simulink model "project2_sim"  (R2021b)
settings: Solver=VariableStepAuto  StartTime=0.0  StopTime=1370
values from neighbouring files (symbols this model uses):
  c0 = 0.1    [project2.m]
  c1 = 0.02    [project2.m]
  cd = 0.3    [project2.m]
  eff = 0.93    [project2.m]
  fuelmap = importdata("FuelMapLookup.csv")    [project2.m]
  G_fd = 3.36    [project2.m]
  Gear_ratio_1 = 4.58    [project2.m]
  Gear_ratio_2 = 2.96    [project2.m]
  Gear_ratio_3 = 1.91    [project2.m]
  Gear_ratio_4 = 1.45    [project2.m]
  Gear_ratio_5 = 1.00    (= 1)    [project2.m]
  Gear_ratio_6 = 0.75    [project2.m]
  input_speed = fuelmapinputs(:,2)    [project2.m]
  input_torques = fuelmapinputs(:,1)    [project2.m]
  Je = 0.1301    [project2.m]
  kd = 0.0    (= 0)    [project2.m]
  kfactor = importdata("k_factor.csv")    [project2.m]
  ki = 0.1    [project2.m]
  kp = 2.86    [project2.m]
  lower_rpm = lower_curve(:,2)    [project2.m]
  lower_torque = lower_curve(:,1)    [project2.m]
  m = (3900*.45359237)    (= 1769.010243)    [project2.m]
  max_break_torque = 375*12*2*3.36    (= 30240)    [project2.m]
  mT = 375    [project2.m]
  r = (0.339)    (= 0.339)    [project2.m]
  rho = 1.225    [project2.m]
  S = 2.3    [project2.m]
  sr = importdata("speed_ratio.csv")    [project2.m]
  time = highway(:,1)    [project2.m]
  tr = importdata("torque_ratio.csv")    [project2.m]
  upper_rpm = upper_curve(:,2)    [project2.m]
  upper_torque = upper_curve(:,1)    [project2.m]
  vel = highway(:,2)    [project2.m]
  w_idle = 720    [project2.m]
  w_max = 6400    [project2.m]
libraries: simulink x2, slpidlib x1
settings Model: Creator=franc  LastModifiedBy=franc

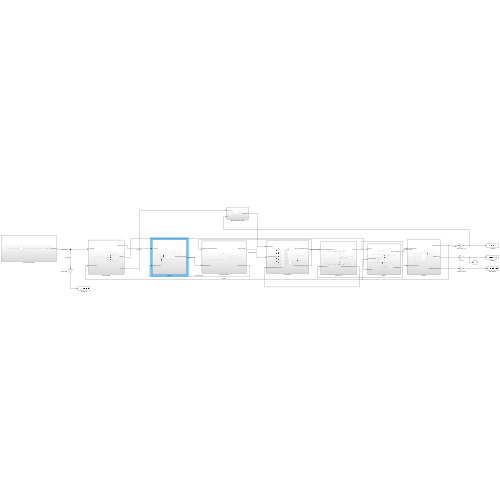
[thumbnail: Simulink's stored preview of the top-level diagram]
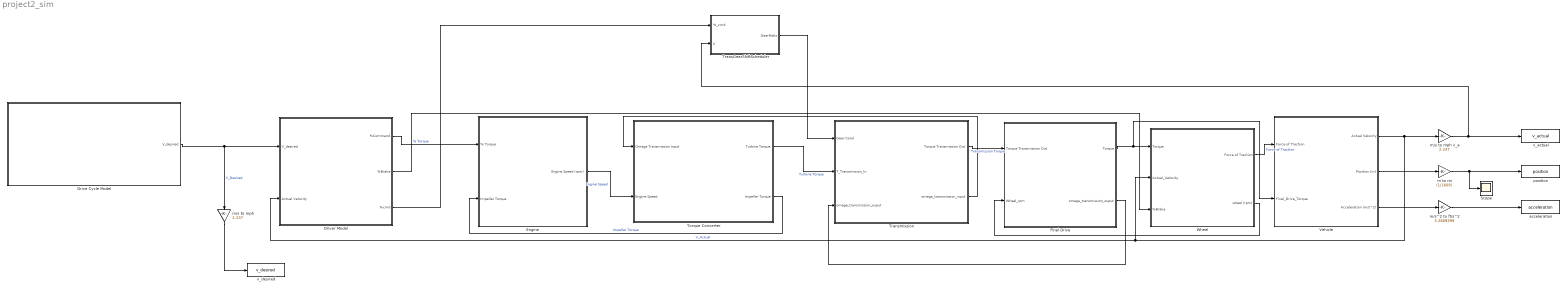
== system project2_sim ==
  " Engine" : Subsystem
  Drive Cycle Model : Subsystem
  Driver Model : Subsystem
  FInal Drive : Subsystem
  Scope : Scope
  Torque Converter : Subsystem
  TransGearShiftScheduler : Subsystem
  Transmission : Subsystem
  Vehicle : Subsystem
  Wheel : Subsystem
  acceleration : ToWorkspace  VariableName=acceleration  SaveFormat=Timeseries  SampleTime=-1
  m to mi : Gain  Gain=(1/1609)
  m/s to mph : Gain  Gain=2.237
  m/s to mph v_a : Gain  Gain=2.237
  m/s^2 to ft/s^2 : Gain  Gain=3.2808399
  position : ToWorkspace  VariableName=position  SaveFormat=Timeseries  SampleTime=-1
  v_actual : ToWorkspace  VariableName=v_actual  SaveFormat=Timeseries  SampleTime=-1
  v_desired : ToWorkspace  VariableName=v_desired  SaveFormat=Timeseries  SampleTime=-1
  wires:
  m/s to mph/1 -> v_desired/1
  m/s^2 to ft/s^2/1 -> acceleration/1
  Vehicle/1(Actual Velocity) -> Driver Model/2(Actual Velocity), Wheel/2(Actual_Velocity), m/s to mph v_a/1  "V_Actual"
  Drive Cycle Model/1(V_desired) -> m/s to mph/1, Driver Model/1(V_desired)  "V_Desired"
  Wheel/1(Force of Traction) -> Vehicle/1(Force of Traction)  "Force of Traction"
  Vehicle/2(Position (m)) -> m to mi/1
  Vehicle/3(Acceleration (m/s^2)) -> m/s^2 to ft/s^2/1
  m to mi/1 -> Scope/1, position/1
  Driver Model/1(%Command) -> " Engine"/1(% Torque)  "% Torque"
  Torque Converter/1(Turbine Torque) -> Transmission/2(T_Transmission_In)  "Turbine Torque"
  Transmission/2(omega_transmission_input) -> Torque Converter/1(Omega Transmission Input)
  Torque Converter/2(Impeller Torque) -> " Engine"/2(Impeller Torque)  "Impeller Torque"
  " Engine"/1(Engine Speed (rpm)) -> Torque Converter/2(Engine Speed)  "Engine Speed"
  m/s to mph v_a/1 -> TransGearShiftScheduler/2(V), v_actual/1
  TransGearShiftScheduler/1(GearRatio) -> Transmission/1(Gear Cond)
  Driver Model/2(%Brake) -> Wheel/3(%Brake)
  Driver Model/3(%cmd) -> TransGearShiftScheduler/1("%_cmd ")
  Transmission/1(Torque Transmission Out) -> FInal Drive/1(Torque Transmission Out)  "Transmission Torque"
  Wheel/2(wheel (rpm)) -> FInal Drive/2(Wheel_rpm)
  FInal Drive/2(omega_transmission_ouput) -> Transmission/3(omega_transmission_ouput)
  FInal Drive/1(Torque) -> Wheel/1(Torque), Vehicle/2(Final_Drive_Torque)

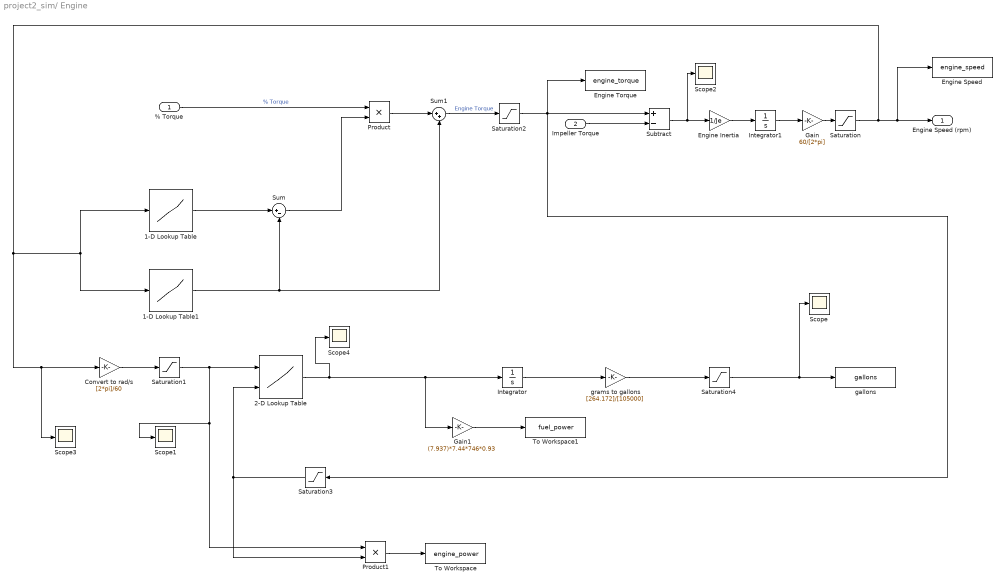
== system project2_sim/ Engine ==
  % Torque : Inport
  Impeller Torque : Inport  Port=2
  1-D Lookup Table : Lookup_n-D  NumberOfTableDimensions=1  BreakpointsForDimension1=upper_rpm  Table=upper_torque  InternalRulePriority=Speed  RndMeth=Simplest  InputSameDT=on
  1-D Lookup Table1 : Lookup_n-D  NumberOfTableDimensions=1  BreakpointsForDimension1=lower_rpm  Table=lower_torque  InternalRulePriority=Speed  RndMeth=Simplest  InputSameDT=on
  2-D Lookup Table : Lookup_n-D  BreakpointsForDimension1=input_speed  BreakpointsForDimension2=input_torques  Table=[fuelmap]  InternalRulePriority=Speed  RndMeth=Simplest  InputSameDT=on
      settings: InputPortMap=u0,u1
  Convert to rad/s : Gain  Gain=[2*pi]/60
  Engine Inertia : Gain  Gain=1/Je
  Engine Speed : ToWorkspace  VariableName=engine_speed  SaveFormat=Timeseries  SampleTime=-1
  Engine Torque : ToWorkspace  VariableName=engine_torque  SaveFormat=Timeseries  SampleTime=-1
  Gain : Gain  Gain=60/[2*pi]
  Gain1 : Gain  Gain=(7.937)*7.44*746*0.93
  Integrator : Integrator
  Integrator1 : Integrator  InitialCondition=w_idle
  Product : Product
  Product1 : Product
  Saturation : Saturate  UpperLimit=w_max  LowerLimit=w_idle
  Saturation1 : Saturate  UpperLimit=706.3  LowerLimit=0
  Saturation2 : Saturate  UpperLimit=mT  LowerLimit=0
  Saturation3 : Saturate  UpperLimit=387.4  LowerLimit=-49.3
  Saturation4 : Saturate  UpperLimit=0.35  LowerLimit=0  ZeroCross=off
  Scope{,1..4} (5 alike) : Scope
  Subtract : Sum  Inputs=+-
  Sum : Sum  Inputs=|+-
  Sum1 : Sum  Inputs=|++
  To Workspace : ToWorkspace  VariableName=engine_power  SaveFormat=Timeseries  SampleTime=-1
  To Workspace1 : ToWorkspace  VariableName=fuel_power  SaveFormat=Timeseries  SampleTime=-1
  gallons : ToWorkspace  VariableName=gallons  SaveFormat=Timeseries  SampleTime=-1
  grams to gallons : Gain  Gain=[264.172]/[105000]
  Engine Speed (rpm) : Outport
  wires:
  % Torque/1 -> Product/1  "% Torque"
  Product/1 -> Sum1/1
  Sum/1 -> Product/2
  1-D Lookup Table/1 -> Sum/1
  1-D Lookup Table1/1 -> Sum1/2, Sum/2
  Sum1/1 -> Saturation2/1  "Engine Torque"
  Saturation/1 -> 1-D Lookup Table/1, 1-D Lookup Table1/1, Scope3/1, Convert to rad/s/1, Engine Speed/1, Engine Speed (rpm)/1
  Impeller Torque/1 -> Subtract/2
  Subtract/1 -> Scope2/1, Engine Inertia/1
  Engine Inertia/1 -> Integrator1/1
  Integrator1/1 -> Gain/1
  Gain/1 -> Saturation/1
  Convert to rad/s/1 -> Saturation1/1
  Saturation2/1 -> Engine Torque/1, Saturation3/1, Subtract/1
  Product1/1 -> To Workspace/1
  2-D Lookup Table/1 -> Scope4/1, Gain1/1, Integrator/1
  Integrator/1 -> grams to gallons/1
  Saturation1/1 -> Scope1/1, Product1/1, 2-D Lookup Table/1
  Saturation3/1 -> 2-D Lookup Table/2, Product1/2
  grams to gallons/1 -> Saturation4/1
  Saturation4/1 -> Scope/1, gallons/1
  Gain1/1 -> To Workspace1/1

== system project2_sim/Drive Cycle Model ==
  1-D Lookup Table : Lookup_n-D  NumberOfTableDimensions=1  BreakpointsForDimension1=time  Table=vel  InternalRulePriority=Speed  RndMeth=Simplest  InputSameDT=on
  Clock : Clock
  mph to m/s : Gain  Gain=(1/2.237)
  V_desired : Outport
  wires:
  1-D Lookup Table/1 -> mph to m/s/1  "V_desired (mph)"
  mph to m/s/1 -> V_desired/1  "V_Desired (m/s)"
  Clock/1 -> 1-D Lookup Table/1

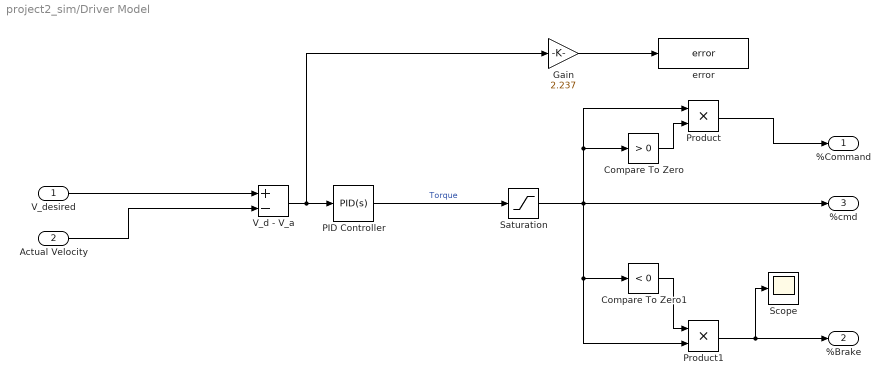
== system project2_sim/Driver Model ==
  V_desired : Inport
  Actual Velocity : Inport  Port=2
  Compare To Zero : simulink/Logic and Bit Operations/Compare To Zero  relop=>  OutDataTypeStr=boolean  ZeroCross=off
  Compare To Zero1 : simulink/Logic and Bit Operations/Compare To Zero  relop=<  OutDataTypeStr=boolean  ZeroCross=off
  Gain : Gain  Gain=2.237
  PID Controller : slpidlib/PID Controller  Controller=PID  Form=Parallel  TimeDomain=Continuous-time  UseExternalTs=off  SampleTime=-1  IntegratorMethod=Forward Euler  FilterMethod=Forward Euler  ControllerParametersSource=internal  P=kp  I=ki  D=kd  UseFilter=on  N=100  TunerSelectOption=Transfer Function Based (PID Tuner App)  InitialConditionSource=internal  InitialConditionForIntegrator=0  InitialConditionForFilter=0  DifferentiatorICPrevScaledInput=0  ExternalReset=none  TrackingMode=off  Kt=1  LimitOutput=off  SatLimitsSource=internal  UpperSaturationLimit=inf  LowerSaturationLimit=-inf  LinearizeAsGain=on  AntiWindupMode=none  Kb=1  POutMin=[]  POutMax=[]  IOutMin=[]  IOutMax=[]  DOutMin=[]  DOutMax=[]  NOutMin=[]  NOutMax=[]  SumOutMin=[]  SumOutMax=[]  SaturationOutMin=[]  SaturationOutMax=[]  PParamMin=[]  PParamMax=[]  IParamMin=[]  IParamMax=[]  DParamMin=[]  DParamMax=[]  NParamMin=[]  NParamMax=[]  KbParamMin=[]  KbParamMax=[]  KtParamMin=[]  KtParamMax=[]  KbOutMin=[]  KbOutMax=[]  KtOutMin=[]  KtOutMax=[]  IntegratorOutMin=[]  IntegratorOutMax=[]  FilterOutMin=[]  FilterOutMax=[]  SumI1OutMin=[]  SumI1OutMax=[]  SumI2OutMin=[]  SumI2OutMax=[]  SumI3OutMin=[]  SumI3OutMax=[]  SumI4OutMin=[]  SumI4OutMax=[]  SumDOutMin=[]  SumDOutMax=[]  DifferentiatorOutMin=[]  DifferentiatorOutMax=[]  FilterDiffOutCoefMin=[]  FilterDiffOutCoefMax=[]  ReciprocalOutMin=[]  ReciprocalOutMax=[]  SumDenOutMin=[]  SumDenOutMax=[]  SumNumOutMin=[]  SumNumOutMax=[]  DivideOutMin=[]  DivideOutMax=[]  UdiffTsProdOutMin=[]  UdiffTsProdOutMax=[]  NTsProdOutMin=[]  NTsProdOutMax=[]  UintegralTsProdOutMin=[]  UintegralTsProdOutMax=[]  UngainTsProdOutMin=[]  UngainTsProdOutMax=[]  IntegratorContinuousStateAttributes=''  IntegratorStateMustResolveToSignalObject=off  IntegratorRTWStateStorageClass=Auto  FilterContinuousStateAttributes=''  FilterStateMustResolveToSignalObject=off  FilterRTWStateStorageClass=Auto  ParallelPVariant=InternalParameters  IdealPVariant=Disabled  IVariant=InternalParameters  DVariant=InternalParameters  IntegratorVariant=Continuous  SatVariant=Disabled  AWVariant=Passthrough  PCopyVariant=Disabled  TRVariant=Disabled  FdbkBlocksVariant=Forward  IdealPFdbkVariant=Disabled  SatFdbkVariant=Disabled  DerivativeFilterVariant=ContFilter  NVariant=InternalParameters  NCopyVariant=Disabled  FilterICVariant=InternalICsFilter  IntegratorICVariant=InternalICs  ExternalResetVariant=Disabled  TRSumVariant=Passthrough  SumFdbkVariant=Disabled  SumVariant=Sum_PID  TsampFilterVariant=InternalTs  TsampNgainVariant=Passthrough  TsampIntegralVariant=Passthrough  ExternalSaturationOutDataTypeStr=Inherit: Same as second input
  Product : Product
  Product1 : Product
  Saturation : Saturate  UpperLimit=1  LowerLimit=-1
  Scope : Scope
  V_d - V_a : Sum  Inputs=+-
  error : ToWorkspace  VariableName=error  SaveFormat=Timeseries  SampleTime=-1
  %Command : Outport
  %Brake : Outport  Port=2
  %cmd : Outport  Port=3
  wires:
  Actual Velocity/1 -> V_d - V_a/2
  V_desired/1 -> V_d - V_a/1
  V_d - V_a/1 -> Gain/1, PID Controller/1
  PID Controller/1 -> Saturation/1  "Torque"
  Gain/1 -> error/1
  Saturation/1 -> %cmd/1, Compare To Zero/1, Product/1, Compare To Zero1/1, Product1/2
  Compare To Zero/1 -> Product/2
  Product/1 -> %Command/1
  Compare To Zero1/1 -> Product1/1
  Product1/1 -> Scope/1, %Brake/1

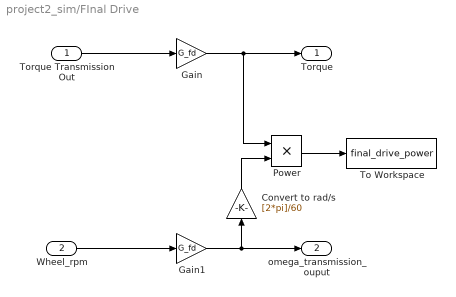
== system project2_sim/FInal Drive ==
  Torque Transmission Out : Inport
  Wheel_rpm : Inport  Port=2
  Convert to rad/s : Gain  Gain=[2*pi]/60
  Gain : Gain  Gain=G_fd
  Gain1 : Gain  Gain=G_fd
  Power : Product
  To Workspace : ToWorkspace  VariableName=final_drive_power  SaveFormat=Timeseries  SampleTime=-1
  Torque : Outport
  omega_transmission_ouput : Outport  Port=2
  wires:
  Torque Transmission Out/1 -> Gain/1
  Gain/1 -> Power/1, Torque/1
  Gain1/1 -> omega_transmission_ouput/1, Convert to rad/s/1
  Wheel_rpm/1 -> Gain1/1
  Power/1 -> To Workspace/1
  Convert to rad/s/1 -> Power/2

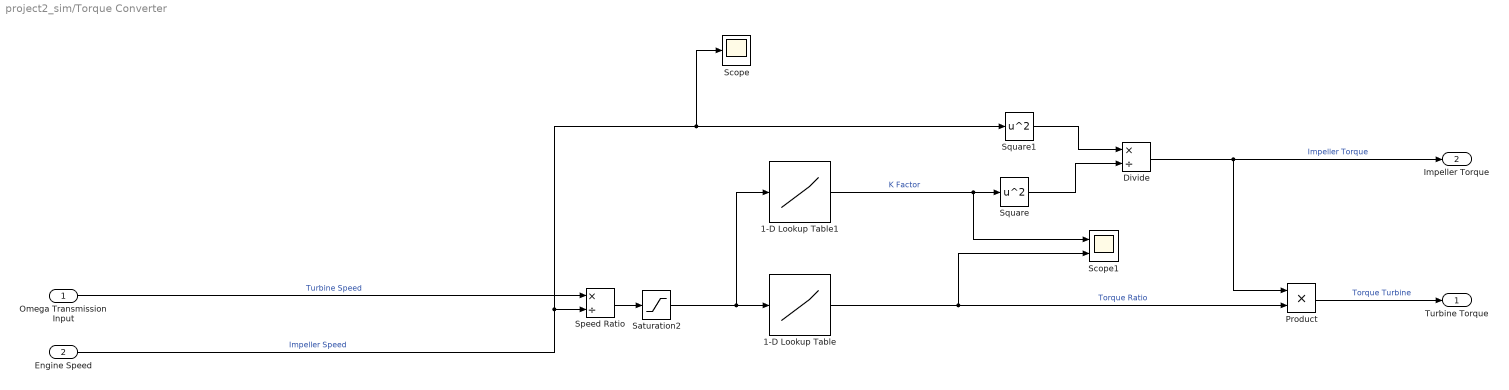
== system project2_sim/Torque Converter ==
  Omega Transmission Input : Inport
  Engine Speed : Inport  Port=2
  1-D Lookup Table : Lookup_n-D  NumberOfTableDimensions=1  BreakpointsForDimension1=sr  Table=tr  InternalRulePriority=Speed  RndMeth=Simplest  InputSameDT=on
  1-D Lookup Table1 : Lookup_n-D  NumberOfTableDimensions=1  BreakpointsForDimension1=sr  Table=kfactor  InternalRulePriority=Speed  RndMeth=Simplest  InputSameDT=on
  Divide : Product  Inputs=*/
  Product : Product
  Saturation2 : Saturate  UpperLimit=1  LowerLimit=0
  Scope : Scope
  Scope1 : Scope  NumInputPorts=2
  Speed Ratio : Product  Inputs=*/
  Square : Math  Operator=square  SaturateOnIntegerOverflow=on
  Square1 : Math  Operator=square  SaturateOnIntegerOverflow=on
  Turbine Torque : Outport
  Impeller Torque : Outport  Port=2
  wires:
  Omega Transmission Input/1 -> Speed Ratio/1  "Turbine Speed"
  Engine Speed/1 -> Scope/1, Square1/1, Speed Ratio/2  "Impeller Speed"
  Speed Ratio/1 -> Saturation2/1
  1-D Lookup Table1/1 -> Scope1/1, Square/1  "K Factor"
  Square1/1 -> Divide/1
  Square/1 -> Divide/2
  1-D Lookup Table/1 -> Scope1/2, Product/2  "Torque Ratio"
  Divide/1 -> Impeller Torque/1, Product/1  "Impeller Torque"
  Product/1 -> Turbine Torque/1  "Torque Turbine"
  Saturation2/1 -> 1-D Lookup Table1/1, 1-D Lookup Table/1

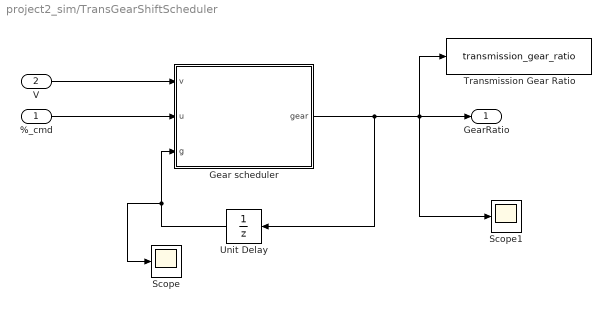
== system project2_sim/TransGearShiftScheduler ==
  "%_cmd " : Inport
  V : Inport  Port=2
  "Gear scheduler " : MATLAB Function  TreatAsAtomicUnit=on
  Scope : Scope
  Scope1 : Scope
  Transmission Gear Ratio : ToWorkspace  VariableName=transmission_gear_ratio  SaveFormat=Timeseries  SampleTime=-1
  Unit Delay : UnitDelay  InitialCondition=1  SampleTime=-1  HasFrameUpgradeWarning=on
  GearRatio : Outport
  wires:
  "Gear scheduler "/1(gear) -> Scope1/1, Transmission Gear Ratio/1, GearRatio/1, Unit Delay/1
  "%_cmd "/1 -> "Gear scheduler "/2(u)
  Unit Delay/1 -> Scope/1, "Gear scheduler "/3(g)
  V/1 -> "Gear scheduler "/1(v)

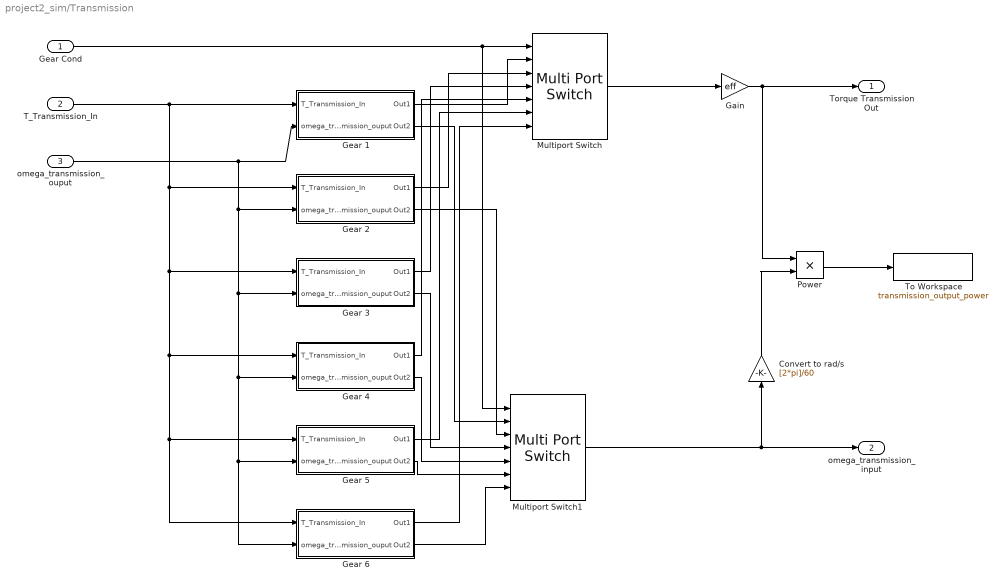
== system project2_sim/Transmission ==
  Gear Cond : Inport
  T_Transmission_In : Inport  Port=2
  omega_transmission_ouput : Inport  Port=3
  Convert to rad/s : Gain  Gain=[2*pi]/60
  Gain : Gain  Gain=eff
  Gear 1 : Subsystem
  Gear 2 : Subsystem
  Gear 3 : Subsystem
  Gear 4 : Subsystem
  Gear 5 : Subsystem
  Gear 6 : Subsystem
  Multiport Switch : MultiPortSwitch  Inputs=6  DiagnosticForDefault=None
  Multiport Switch1 : MultiPortSwitch  Inputs=6  DiagnosticForDefault=None
  Power : Product
  To Workspace : ToWorkspace  VariableName=transmission_output_power  SaveFormat=Timeseries  SampleTime=-1
  Torque Transmission Out : Outport
  omega_transmission_input : Outport  Port=2
  wires:
  Gear Cond/1 -> Multiport Switch1/1, Multiport Switch/1
  T_Transmission_In/1 -> Gear 1/1(T_Transmission_In), Gear 2/1(T_Transmission_In), Gear 3/1(T_Transmission_In), Gear 4/1(T_Transmission_In), Gear 5/1(T_Transmission_In), Gear 6/1(T_Transmission_In)
  omega_transmission_ouput/1 -> Gear 2/2(omega_transmission_ouput), Gear 3/2(omega_transmission_ouput), Gear 4/2(omega_transmission_ouput), Gear 5/2(omega_transmission_ouput), Gear 6/2(omega_transmission_ouput), Gear 1/2(omega_transmission_ouput)
  Gear 1/1(Out1) -> Multiport Switch/2
  Gear 2/1(Out1) -> Multiport Switch/3
  Gear 3/1(Out1) -> Multiport Switch/4
  Gear 4/1(Out1) -> Multiport Switch/5
  Gear 5/1(Out1) -> Multiport Switch/6
  Gear 6/1(Out1) -> Multiport Switch/7
  Gear 1/2(Out2) -> Multiport Switch1/2
  Gear 2/2(Out2) -> Multiport Switch1/3
  Gear 3/2(Out2) -> Multiport Switch1/4
  Gear 4/2(Out2) -> Multiport Switch1/5
  Gear 5/2(Out2) -> Multiport Switch1/6
  Gear 6/2(Out2) -> Multiport Switch1/7
  Gain/1 -> Torque Transmission Out/1, Power/1
  Multiport Switch/1 -> Gain/1
  Multiport Switch1/1 -> Convert to rad/s/1, omega_transmission_input/1
  Convert to rad/s/1 -> Power/2
  Power/1 -> To Workspace/1

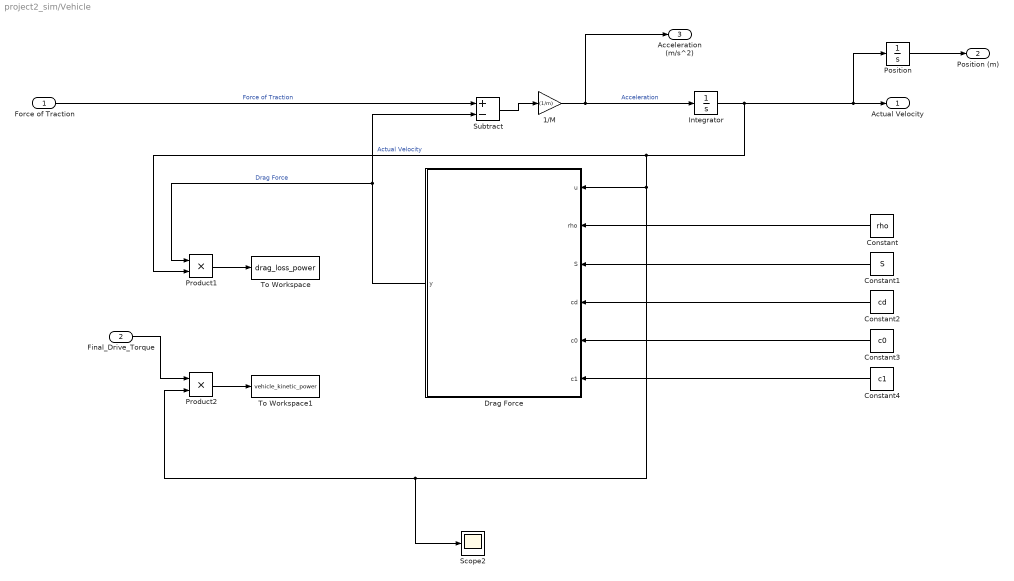
== system project2_sim/Vehicle ==
  Force of Traction : Inport
  Final_Drive_Torque : Inport  Port=2
  1/M : Gain  Gain=(1/m)
  Constant : Constant  Value=rho
  Constant1 : Constant  Value=S
  Constant2 : Constant  Value=cd
  Constant3 : Constant  Value=c0
  Constant4 : Constant  Value=c1
  Drag Force : MATLAB Function  TreatAsAtomicUnit=on
  Integrator : Integrator  InitialCondition=0.0001
  Position : Integrator
  Product1 : Product
  Product2 : Product
  Scope2 : Scope
  Subtract : Sum  Inputs=+-
  To Workspace : ToWorkspace  VariableName=drag_loss_power  SaveFormat=Timeseries  SampleTime=-1
  To Workspace1 : ToWorkspace  VariableName=vehicle_kinetic_power  SaveFormat=Timeseries  SampleTime=-1
  Actual Velocity : Outport
  Position (m) : Outport  Port=2
  Acceleration (m/s^2) : Outport  Port=3
  wires:
  Force of Traction/1 -> Subtract/1  "Force of Traction"
  1/M/1 -> Acceleration (m/s^2)/1, Integrator/1  "Acceleration"
  Integrator/1 -> Product1/2, Product2/2, Scope2/1, Drag Force/1(u), Position/1, Actual Velocity/1  "Actual Velocity"
  Subtract/1 -> 1/M/1
  Drag Force/1(y) -> Product1/1, Subtract/2  "Drag Force"
  Constant/1 -> Drag Force/2(rho)
  Constant1/1 -> Drag Force/3(S)
  Constant2/1 -> Drag Force/4(cd)
  Constant3/1 -> Drag Force/5(c0)
  Constant4/1 -> Drag Force/6(c1)
  Position/1 -> Position (m)/1
  Product1/1 -> To Workspace/1
  Product2/1 -> To Workspace1/1
  Final_Drive_Torque/1 -> Product2/1

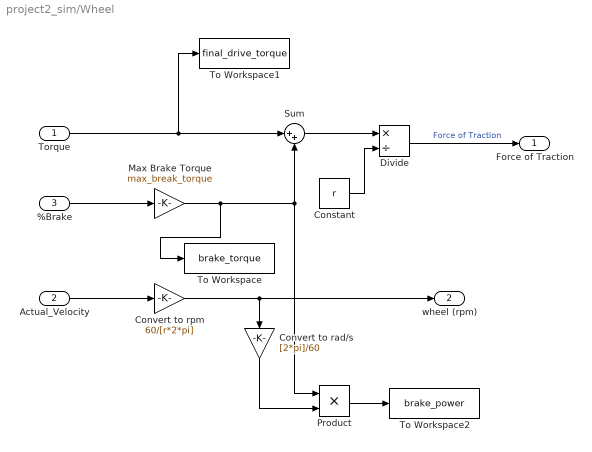
== system project2_sim/Wheel ==
  Torque : Inport
  Actual_Velocity : Inport  Port=2
  %Brake : Inport  Port=3
  Constant : Constant  Value=r
  Convert to rad/s : Gain  Gain=[2*pi]/60
  Convert to rpm : Gain  Gain=60/[r*2*pi]
  Divide : Product  Inputs=*/
  Max Brake Torque : Gain  Gain=max_break_torque
  Product : Product
  Sum : Sum  Inputs=|++
  To Workspace : ToWorkspace  VariableName=brake_torque  SaveFormat=Timeseries  SampleTime=-1
  To Workspace1 : ToWorkspace  VariableName=final_drive_torque  SaveFormat=Timeseries  SampleTime=-1
  To Workspace2 : ToWorkspace  VariableName=brake_power  SaveFormat=Timeseries  SampleTime=-1
  Force of Traction : Outport
  wheel (rpm) : Outport  Port=2
  wires:
  Divide/1 -> Force of Traction/1  "Force of Traction"
  Constant/1 -> Divide/2
  Actual_Velocity/1 -> Convert to rpm/1
  Convert to rpm/1 -> Convert to rad/s/1, wheel (rpm)/1
  %Brake/1 -> Max Brake Torque/1
  Sum/1 -> Divide/1
  Torque/1 -> Sum/1, To Workspace1/1
  Max Brake Torque/1 -> To Workspace/1, Sum/2, Product/1
  Convert to rad/s/1 -> Product/2
  Product/1 -> To Workspace2/1

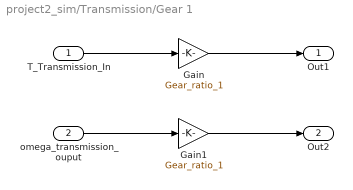
== system project2_sim/Transmission/Gear 1 ==
  T_Transmission_In : Inport
  omega_transmission_ouput : Inport  Port=2
  Gain : Gain  Gain=Gear_ratio_1
  Gain1 : Gain  Gain=Gear_ratio_1
  Out1 : Outport
  Out2 : Outport  Port=2
  wires:
  T_Transmission_In/1 -> Gain/1
  Gain/1 -> Out1/1
  omega_transmission_ouput/1 -> Gain1/1
  Gain1/1 -> Out2/1

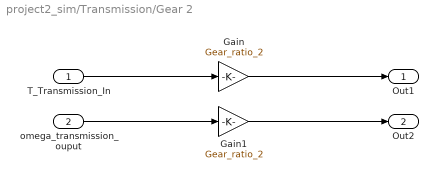
== system project2_sim/Transmission/Gear 2 ==
  T_Transmission_In : Inport
  omega_transmission_ouput : Inport  Port=2
  Gain : Gain  Gain=Gear_ratio_2
  Gain1 : Gain  Gain=Gear_ratio_2
  Out1 : Outport
  Out2 : Outport  Port=2
  wires:
  T_Transmission_In/1 -> Gain/1
  Gain/1 -> Out1/1
  omega_transmission_ouput/1 -> Gain1/1
  Gain1/1 -> Out2/1

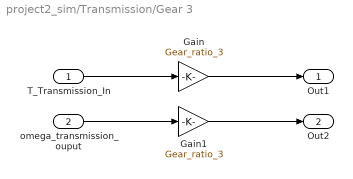
== system project2_sim/Transmission/Gear 3 ==
  T_Transmission_In : Inport
  omega_transmission_ouput : Inport  Port=2
  Gain : Gain  Gain=Gear_ratio_3
  Gain1 : Gain  Gain=Gear_ratio_3
  Out1 : Outport
  Out2 : Outport  Port=2
  wires:
  T_Transmission_In/1 -> Gain/1
  Gain/1 -> Out1/1
  omega_transmission_ouput/1 -> Gain1/1
  Gain1/1 -> Out2/1

== system project2_sim/Transmission/Gear 4 ==
  T_Transmission_In : Inport
  omega_transmission_ouput : Inport  Port=2
  Gain : Gain  Gain=Gear_ratio_4
  Gain1 : Gain  Gain=Gear_ratio_4
  Out1 : Outport
  Out2 : Outport  Port=2
  wires:
  T_Transmission_In/1 -> Gain/1
  Gain/1 -> Out1/1
  omega_transmission_ouput/1 -> Gain1/1
  Gain1/1 -> Out2/1

== system project2_sim/Transmission/Gear 5 ==
  T_Transmission_In : Inport
  omega_transmission_ouput : Inport  Port=2
  Gain : Gain  Gain=Gear_ratio_5
  Gain1 : Gain  Gain=Gear_ratio_5
  Out1 : Outport
  Out2 : Outport  Port=2
  wires:
  T_Transmission_In/1 -> Gain/1
  Gain/1 -> Out1/1
  omega_transmission_ouput/1 -> Gain1/1
  Gain1/1 -> Out2/1

== system project2_sim/Transmission/Gear 6 ==
  T_Transmission_In : Inport
  omega_transmission_ouput : Inport  Port=2
  Gain : Gain  Gain=Gear_ratio_6
  Gain1 : Gain  Gain=Gear_ratio_6
  Out1 : Outport
  Out2 : Outport  Port=2
  wires:
  T_Transmission_In/1 -> Gain/1
  Gain/1 -> Out1/1
  omega_transmission_ouput/1 -> Gain1/1
  Gain1/1 -> Out2/1

== matlab function project2_sim/Vehicle/Drag Force ==
  data: u input; y output; rho input; S input; cd input; c0 input; c1 input
function y = fcn(u,rho,S,cd,c0,c1)
c2 = 0.5*(rho)*(S)*(cd);
fDrag = (c0 - c1*u - c2*(u)^2);
y = fDrag;

== matlab function project2_sim/TransGearShiftScheduler/Gear scheduler  ==
  data: v input; gear output; u input; g input
function gear = fcn(v,u,g)
if u>0
    if (v<12.3*0.44704)
        gear = 1;
    elseif (v>=12.3*0.44704 && v<24.6*0.44704 && g==1)
        gear = 2;
    elseif (v>=24.6*0.44704 && v<35.79*0.44704 && g==2)
        gear = 3;
    elseif (v>=35.8*0.44704 && v<46.9*0.44704 && g==3)
        gear = 4;
    elseif (v>46.9*0.44704 && v<80*0.44704 && g==4)
        gear = 5;
    elseif (v>80*0.44704 && g==5)
        gear = 6;
    else
        gear = g;
    end
    
elseif u<=0
    if (v>78*0.44704)
        gear = 6;
    elseif (v<=78*0.44704 && v>43*0.44704 && g == 6)
        gear = 5;
    elseif (v<=43*0.44704 && v>32*0.44704 && g == 5)
        gear = 4;
    elseif (v<=32*0.44704 && v>23*0.44704 && g == 4)
        gear = 3;
    elseif (v<=23*0.44704 && v>10*0.44704 && g ==3)
        gear = 2;
    elseif (v<10*0.44704 && g == 2)
     gear = 1;
    else
        gear = g;
    end
else
    gear = g;
    

end
